simulink model "Cardiovascular"  (Simulink 6.4)
settings: Solver=ode45  StartTime=0.0  StopTime=50  MaxStep=0.01  MinStep=0.0000000000001  RelTol=1e-1
values from neighbouring files (symbols this model uses):
  A = 20.9    [Gas_Exchange_IC.m]    (also in getPneumonia.m = (LF1-LF2)/(1-exp(Rresolve*(t2(end)-t2(1)))))
  B = 92.8    [Gas_Exchange_IC.m]    (also in getPneumonia.m = LungFunction(end)-A)
  C = 10570    [Gas_Exchange_IC.m]
  D = -5.251    [Gas_Exchange_IC.m]
  fcs_max = 47.78    [Cardiovascular_IC.m]    (also in Reflex_Ursino_IC.m)
  fcs_min = 2.52    [Cardiovascular_IC.m]    (also in Reflex_Ursino_IC.m)
  ftbs_min = 0.1    [Cardiovascular_IC.m]    (also in SA_Node_Ursino_IC.m)
  HP_basal = 0.58    [Cardiovascular_IC.m]    (also in SA_Node_Ursino_IC.m)
  k_cs = 11.758    [Cardiovascular_IC.m]    (also in Reflex_Ursino_IC.m)
  Pn = 90    [Cardiovascular_IC.m]    (also in Reflex_Ursino_IC.m)
undefined symbols (not defined in the file or in its folder): Cbp, Cbv, Cep, Cev, Chp, Chv, Cla, Cmp, Cmv, Cpa, Cpp, Cpv, Cra, Csa, Csp, Csv, CvbO2_n, CvhO2_n, CvmO2_n, Dx, ftas_min, Gas_sleep, GbO2, Gbs_sleep, GhO2, GmO2, Gpara_sleep, initx, k_cs_sleep, KElv, KErv, KhCO2, KmCO2, Kr_vc, KRlv, KRrv, ksys, Lpa, Lsa, Mb, Mhn, Mm, P0lv, P0rv, PaCO2_n, Pn_sleep, R_vc_0, Rbpn, Rbv, Rev, Rhpn, Rhv, Rla, Rmv, Rpa, Rpp, Rpv, Rra, Rsa, Rsv ... (+25)
(part 2 of 2)

== system Cardiovascular/Systemic/Systemic  Arteries ==
  Qlv : Inport
  Constant2 : Constant  Value=Vusa  OutDataType=sfix(16)  ConRadixGroup=Use specified scaling  OutScaling=2^0  SampleTime=inf  FramePeriod=inf
  Gain : Gain  Gain=1/Csa  SaturateOnIntegerOverflow=on
  Gain1 : Gain  Orientation=left  Gain=1/Lsa  SaturateOnIntegerOverflow=on
  Gain2 : Gain  Gain=Rsa  SaturateOnIntegerOverflow=on
  Integrator : Integrator  InitialCondition=25.863
  Integrator1 : Integrator  Orientation=left
  SubSystem : Subsystem
  Sum : Sum  Inputs=|+-
  Sum1 : Sum  Inputs=+-  SaturateOnIntegerOverflow=on  InputSameDT=on
  Sum2 : Sum  Inputs=-+-  SaturateOnIntegerOverflow=on  InputSameDT=on
  Qsa : Outport
  tag scope: ABP=global, Vsa=scoped
  wires:
  Sum1/1 -> Integrator/1
  Integrator1/1 -> Gain1/1
  Sum2/1 -> Integrator1/1
  Gain2/1 -> Sum2/3
  Gain1/1 -> Sum1/2, Gain2/1, Qsa/1  "Qsa"
  Integrator/1 -> SubSystem/2(+)
  SubSystem/1(Out) -> Gain/1, [Vsa]
  Constant2/1 -> SubSystem/1(_)
  Qlv/1 -> Sum1/1
  [Psp] -> Sum2/1
  [gPpl] -> Sum/2
  Gain/1 -> Sum/1, [ABP]  "Psa"
  Sum/1 -> Sum2/2

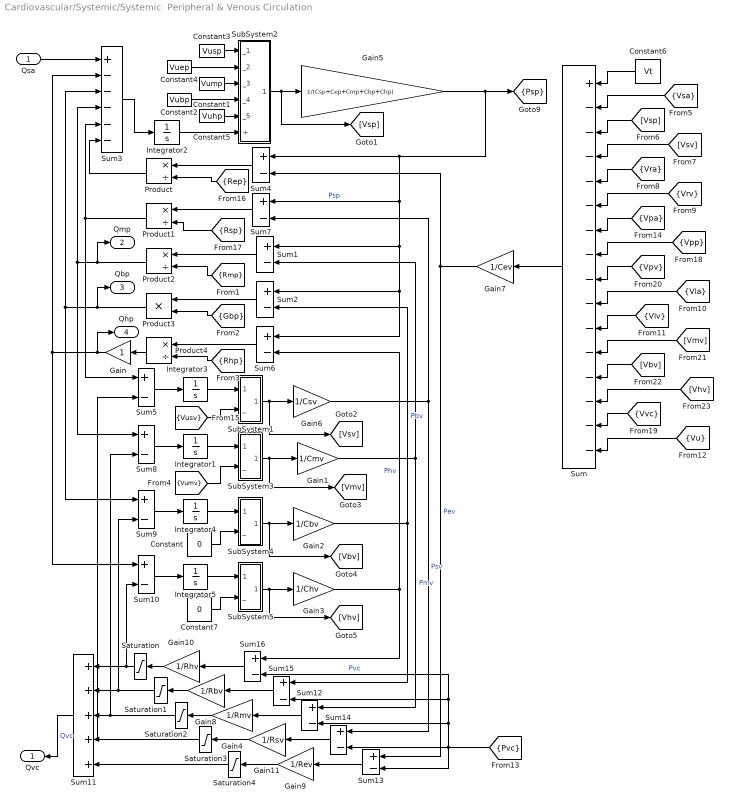
== system Cardiovascular/Systemic/Systemic  Peripheral & Venous Circulation ==
  Qsa : Inport
  Constant : Constant  Value=0  OutDataType=sfix(16)  ConRadixGroup=Use specified scaling  OutScaling=2^0  SampleTime=inf  FramePeriod=inf
  Constant1 : Constant  Value=Vump  OutDataType=sfix(16)  ConRadixGroup=Use specified scaling  OutScaling=2^0  SampleTime=inf  FramePeriod=inf
  Constant2 : Constant  Value=Vubp  OutDataType=sfix(16)  ConRadixGroup=Use specified scaling  OutScaling=2^0  SampleTime=inf  FramePeriod=inf
  Constant3 : Constant  Value=Vusp  OutDataType=sfix(16)  ConRadixGroup=Use specified scaling  OutScaling=2^0  SampleTime=inf  FramePeriod=inf
  Constant4 : Constant  Value=Vuep  OutDataType=sfix(16)  ConRadixGroup=Use specified scaling  OutScaling=2^0  SampleTime=inf  FramePeriod=inf
  Constant5 : Constant  Value=Vuhp  OutDataType=sfix(16)  ConRadixGroup=Use specified scaling  OutScaling=2^0  SampleTime=inf  FramePeriod=inf
  Constant6 : Constant  Orientation=left  Value=Vt  OutDataType=sfix(16)  ConRadixGroup=Use specified scaling  OutScaling=2^0  SampleTime=inf  FramePeriod=inf
  Constant7 : Constant  Value=0  OutDataType=sfix(16)  ConRadixGroup=Use specified scaling  OutScaling=2^0  SampleTime=inf  FramePeriod=inf
  Gain : Gain  Orientation=left
  Gain1 : Gain  Gain=1/Cmv  SaturateOnIntegerOverflow=on
  Gain10 : Gain  Orientation=left  Gain=1/Rhv  SaturateOnIntegerOverflow=on
  Gain11 : Gain  Orientation=left  Gain=1/Rsv  SaturateOnIntegerOverflow=on
  Gain2 : Gain  Gain=1/Cbv  SaturateOnIntegerOverflow=on
  Gain3 : Gain  Gain=1/Chv  SaturateOnIntegerOverflow=on
  Gain4 : Gain  Orientation=left  Gain=1/Rmv  SaturateOnIntegerOverflow=on
  Gain5 : Gain  Gain=1/(Csp+Cep+Cmp+Cbp+Chp)  SaturateOnIntegerOverflow=on
  Gain6 : Gain  Gain=1/Csv  SaturateOnIntegerOverflow=on
  Gain7 : Gain  Orientation=left  Gain=1/Cev  SaturateOnIntegerOverflow=on
  Gain8 : Gain  Orientation=left  Gain=1/Rbv  SaturateOnIntegerOverflow=on
  Gain9 : Gain  Orientation=left  Gain=1/Rev  SaturateOnIntegerOverflow=on
  Integrator{1,3..5} (4 alike) : Integrator
  Integrator2 : Integrator  InitialCondition=Vusp + Vuep+Vump+Vubp+Vuhp
  Product{,1..2,4} (4 alike) : Product  Orientation=left  Inputs=*/  SaturateOnIntegerOverflow=on  RndMeth=Zero  InputSameDT=on
  Product3 : Product  Orientation=left  Inputs=**  SaturateOnIntegerOverflow=on  RndMeth=Zero  InputSameDT=on
  Saturation : Saturate  Orientation=left  UpperLimit=10000  LowerLimit=1
  Saturation1 : Saturate  Orientation=left  UpperLimit=10000  LowerLimit=4
  Saturation2 : Saturate  Orientation=left  UpperLimit=10000  LowerLimit=8
  Saturation3 : Saturate  Orientation=left  UpperLimit=10000  LowerLimit=10
  Saturation4 : Saturate  Orientation=left  UpperLimit=10000  LowerLimit=10
  SubSystem1 : Subsystem
  SubSystem2 : Subsystem
  SubSystem3 : Subsystem
  SubSystem4 : Subsystem
  SubSystem5 : Subsystem
  Sum : Sum  Orientation=left  Inputs=+---------------  SaturateOnIntegerOverflow=on  InputSameDT=on
  Sum{1..2,4,6..7,12..16} (10 alike) : Sum  Orientation=left  Inputs=+-  SaturateOnIntegerOverflow=on  InputSameDT=on
  Sum{5,8..10} (4 alike) : Sum  Inputs=+-  SaturateOnIntegerOverflow=on  InputSameDT=on
  Sum11 : Sum  Orientation=left  Inputs=+++++  SaturateOnIntegerOverflow=on  InputSameDT=on
  Sum3 : Sum  Inputs=+-----  SaturateOnIntegerOverflow=on  InputSameDT=on
  Qvc : Outport  Orientation=left
  Qmp : Outport  Port=2
  Qbp : Outport  Port=3
  Qhp : Outport  Port=4
  tag scope: Psp=scoped
  wires:
  Gain5/1 -> Sum4/1, Sum6/1, Sum2/1, Sum1/1, Sum7/1, [Psp]  "Psp"
  Product1/1 -> Sum3/5, Sum5/1
  Integrator3/1 -> SubSystem1/1(+)
  SubSystem1/1(Out) -> Gain6/1, [Vsv]
  Integrator2/1 -> SubSystem2/6(+)
  SubSystem2/1(Out) -> Gain5/1, [Vsp]
  Sum13/1 -> Gain9/1
  Gain9/1 -> Saturation4/1
  Sum14/1 -> Gain11/1
  [Pvc] -> Sum13/2, Sum14/2, Sum12/2, Sum15/2, Sum16/2  "Pvc"
  Sum5/1 -> Integrator3/1
  Gain11/1 -> Saturation3/1
  [Vusv] -> SubSystem1/2(_)
  Constant3/1 -> SubSystem2/1(_1)
  Constant4/1 -> SubSystem2/2(_2)
  Sum4/1 -> Product/1
  [Rep] -> Product/2
  [Rsp] -> Product1/2
  Sum7/1 -> Product1/1
  Gain6/1 -> Sum7/2, Sum14/1  "Psv"
  Qsa/1 -> Sum3/1
  Gain7/1 -> Sum4/2, Sum13/1  "Pev"
  Sum11/1 -> Qvc/1  "Qvc"
  Sum1/1 -> Product2/1
  [Rmp] -> Product2/2
  Sum2/1 -> Product3/1
  [Gbp] -> Product3/2
  Sum6/1 -> Product4/1
  [Rhp] -> Product4/2
  Product4/1 -> Gain/1
  Product3/1 -> Sum3/3, Sum9/1, Qbp/1
  Product2/1 -> Sum3/4, Sum8/1, Qmp/1
  Product/1 -> Sum3/6
  Constant1/1 -> SubSystem2/3(_3)
  Constant2/1 -> SubSystem2/4(_4)
  Constant5/1 -> SubSystem2/5(_5)
  Sum3/1 -> Integrator2/1
  Integrator1/1 -> SubSystem3/1(+)
  SubSystem3/1(Out) -> Gain1/1, [Vmv]
  Sum8/1 -> Integrator1/1
  [Vumv] -> SubSystem3/2(_)
  Constant6/1 -> Sum/1
  [Vsa] -> Sum/2
  [Vsp] -> Sum/3
  [Vsv] -> Sum/4
  [Vra] -> Sum/5
  [Vrv] -> Sum/6
  [Vpa] -> Sum/7
  [Vpp] -> Sum/8
  [Vpv] -> Sum/9
  [Vla] -> Sum/10
  [Vlv] -> Sum/11
  [Vu] -> Sum/16
  [Vvc] -> Sum/15
  Sum/1 -> Gain7/1
  [Vmv] -> Sum/12
  [Vbv] -> Sum/13
  [Vhv] -> Sum/14
  Integrator4/1 -> SubSystem4/1(+)
  SubSystem4/1(Out) -> Gain2/1, [Vbv]
  Sum9/1 -> Integrator4/1
  Constant/1 -> SubSystem4/2(_)
  Integrator5/1 -> SubSystem5/1(+)
  SubSystem5/1(Out) -> Gain3/1, [Vhv]
  Sum10/1 -> Integrator5/1
  Constant7/1 -> SubSystem5/2(_)
  Gain1/1 -> Sum1/2, Sum12/1  "Pmv"
  Gain2/1 -> Sum2/2, Sum15/1  "Pbv"
  Gain3/1 -> Sum6/2, Sum16/1  "Phv"
  Sum12/1 -> Gain4/1
  Gain4/1 -> Saturation2/1
  Sum15/1 -> Gain8/1
  Gain8/1 -> Saturation1/1
  Sum16/1 -> Gain10/1
  Gain10/1 -> Saturation/1
  Gain/1 -> Sum3/2, Sum10/1, Qhp/1
  Saturation/1 -> Sum11/1, Sum10/2
  Saturation1/1 -> Sum11/2, Sum9/2
  Saturation2/1 -> Sum11/3, Sum8/2
  Saturation3/1 -> Sum11/4, Sum5/2
  Saturation4/1 -> Sum11/5

== system Cardiovascular/Systemic/Vena Cava ==
  Qvc : Inport
  Integrator4 : Integrator
  Product2 : Product  Orientation=left  Inputs=*/  SaturateOnIntegerOverflow=on  RndMeth=Zero  InputSameDT=on
  Pvc : Fcn  Expr=(u>=V_vc_0)*(D1+K1_vc*(u-V_vc_0)) + ( u<V_vc_0)*(D2 + K2_vc*exp(u/V_vc_min))
  Rvc : Fcn  Orientation=left  Expr="Kr_vc * (V_vc_max/u)*  (V_vc_max/u) + R_vc_0"
  Saturation : Saturate  Orientation=left  UpperLimit=10000  LowerLimit=0  ZeroCross=off
  SubSystem3 : Subsystem
  Sum10 : Sum  Inputs=+-  SaturateOnIntegerOverflow=on  InputSameDT=on
  Sum12 : Sum  Orientation=left  Inputs=+-  SaturateOnIntegerOverflow=on  InputSameDT=on
  Sum8 : Sum  Inputs=|++
  V_vc_0 : Constant  Value=130  OutDataType=sfix(16)  ConRadixGroup=Use specified scaling  OutScaling=2^0  SampleTime=inf  FramePeriod=inf
  Qra : Outport  Orientation=left
  tag scope: Pvc=scoped, Vvc=scoped
  wires:
  [gPpl] -> Sum8/2
  Integrator4/1 -> SubSystem3/1(+)
  Sum10/1 -> Integrator4/1
  V_vc_0/1 -> SubSystem3/2(_)
  Pvc/1 -> Sum8/1
  SubSystem3/1(Out) -> Pvc/1, [Vvc]
  Sum8/1 -> [Pvc], Sum12/1
  [Vvc] -> Rvc/1
  [Pra] -> Sum12/2
  Sum12/1 -> Product2/1
  Rvc/1 -> Product2/2
  Product2/1 -> Saturation/1  "Qra"
  Qvc/1 -> Sum10/1
  Saturation/1 -> Sum10/2, Qra/1

== system Cardiovascular/TPR Change/Peri Circ Rep ==
  fes : Inport
  Gas(SI) : Inport  Port=2
  Constant : Constant  Value=ftas_min  OutDataType=sfix(16)  ConRadixGroup=Use specified scaling  OutScaling=2^0  SampleTime=inf  FramePeriod=inf
  Constant1 : Constant  Value=initx(4)  OutDataType=sfix(16)  ConRadixGroup=Use specified scaling  OutScaling=2^0  SampleTime=inf  FramePeriod=inf
  Gain1 : Gain  Gain=0.5  SaturateOnIntegerOverflow=on
  Gain_Rep : Gain  Gain=1.94  SaturateOnIntegerOverflow=on
  Math Function : Math  Operator=log  SaturateOnIntegerOverflow=on
  Product3 : Product  SaturateOnIntegerOverflow=on  InputSameDT=on
  Saturation : Saturate  UpperLimit=inf  LowerLimit=1
  Sum : Sum  Inputs=|+-  SaturateOnIntegerOverflow=on  InputSameDT=on
  Sum1 : Sum  SaturateOnIntegerOverflow=on  InputSameDT=on
  Transfer Fcn : TransferFcn  Denominator=[toux(4) 1]
  Transport Delay : TransportDelay  DelayTime=Dx(4)*0.7  InitialOutput=10  BufferSize=19456
  Rep : Outport
  wires:
  Constant1/1 -> Gain1/1
  Sum1/1 -> Rep/1
  Transfer Fcn/1 -> Sum1/1
  Math Function/1 -> Gain_Rep/1
  Saturation/1 -> Math Function/1
  Sum/1 -> Saturation/1
  Constant/1 -> Sum/2
  Transport Delay/1 -> Sum/1
  fes/1 -> Transport Delay/1
  Gas(SI)/1 -> Product3/2
  Gain_Rep/1 -> Product3/1
  Product3/1 -> Transfer Fcn/1
  Gain1/1 -> Sum1/2

== system Cardiovascular/TPR Change/Peri Circ Rmp ==
  fes : Inport
  Gas(SI) : Inport  Port=2
  Constant : Constant  Value=ftas_min  OutDataType=sfix(16)  ConRadixGroup=Use specified scaling  OutScaling=2^0  SampleTime=inf  FramePeriod=inf
  Constant1 : Constant  Value=initx(10)  OutDataType=sfix(16)  ConRadixGroup=Use specified scaling  OutScaling=2^0  SampleTime=inf  FramePeriod=inf
  Gain1 : Gain  Orientation=up  Gain=0.5  SaturateOnIntegerOverflow=on
  Gain_Rmp : Gain  Gain=2.47  SaturateOnIntegerOverflow=on
  Math Function : Math  Operator=log  SaturateOnIntegerOverflow=on
  Product3 : Product  SaturateOnIntegerOverflow=on  InputSameDT=on
  Saturation : Saturate  UpperLimit=inf  LowerLimit=1
  Sum : Sum  Inputs=+-  SaturateOnIntegerOverflow=on  InputSameDT=on
  Sum1 : Sum  SaturateOnIntegerOverflow=on  InputSameDT=on
  Transfer Fcn : TransferFcn  Denominator=[toux(10) 1]
  Transport Delay : TransportDelay  DelayTime=Dx(10)*0.7  InitialOutput=10  BufferSize=19456
  Rmp_n : Outport
  wires:
  Constant1/1 -> Gain1/1
  Sum1/1 -> Rmp_n/1
  Transfer Fcn/1 -> Sum1/1
  Math Function/1 -> Gain_Rmp/1
  Saturation/1 -> Math Function/1
  Sum/1 -> Saturation/1
  Constant/1 -> Sum/2
  Transport Delay/1 -> Sum/1
  fes/1 -> Transport Delay/1
  Gas(SI)/1 -> Product3/2
  Gain_Rmp/1 -> Product3/1
  Product3/1 -> Transfer Fcn/1
  Gain1/1 -> Sum1/2

== system Cardiovascular/TPR Change/Peri Circ Rsp ==
  fes : Inport
  Gas(SI) : Inport  Port=2
  Constant : Constant  Value=ftas_min  OutDataType=sfix(16)  ConRadixGroup=Use specified scaling  OutScaling=2^0  SampleTime=inf  FramePeriod=inf
  Constant1 : Constant  Value=initx(3)  OutDataType=sfix(16)  ConRadixGroup=Use specified scaling  OutScaling=2^0  SampleTime=inf  FramePeriod=inf
  Gain : Gain  Gain=0.5  SaturateOnIntegerOverflow=on
  Gain_Rsp : Gain  Gain=0.695  SaturateOnIntegerOverflow=on
  Math Function : Math  Operator=log  SaturateOnIntegerOverflow=on
  Product3 : Product  SaturateOnIntegerOverflow=on  InputSameDT=on
  Saturation : Saturate  UpperLimit=inf  LowerLimit=1
  Sum : Sum  Inputs=+-  SaturateOnIntegerOverflow=on  InputSameDT=on
  Sum1 : Sum  SaturateOnIntegerOverflow=on  InputSameDT=on
  Transfer Fcn : TransferFcn  Denominator=[toux(3) 1]
  Transport Delay : TransportDelay  DelayTime=Dx(3)*0.7  InitialOutput=10  BufferSize=19456
  Rsp : Outport
  wires:
  fes/1 -> Transport Delay/1
  Transport Delay/1 -> Sum/1
  Constant/1 -> Sum/2
  Sum/1 -> Saturation/1
  Saturation/1 -> Math Function/1
  Math Function/1 -> Gain_Rsp/1
  Transfer Fcn/1 -> Sum1/1
  Sum1/1 -> Rsp/1
  Constant1/1 -> Gain/1
  Gas(SI)/1 -> Product3/2
  Gain_Rsp/1 -> Product3/1
  Product3/1 -> Transfer Fcn/1
  Gain/1 -> Sum1/2

== system Cardiovascular/TPR Change/Saving TPR ==
  In1 : Inport
  Clock : Clock
      settings: Decimation=10
  Gain : Gain  Gain=1/(3600*24*7)
  Rounding Function : Rounding
  Switch Case : SwitchCase  CaseConditions={0,1,2,3,4,5,6,7,8}  SampleTime=0.1
  Switch Case Action Subsystem : Subsystem  TreatAsAtomicUnit=on
  Switch Case Action Subsystem1 : Subsystem  TreatAsAtomicUnit=on
  Switch Case Action Subsystem2 : Subsystem  TreatAsAtomicUnit=on
  Switch Case Action Subsystem3 : Subsystem  TreatAsAtomicUnit=on
  Switch Case Action Subsystem4 : Subsystem  TreatAsAtomicUnit=on
  Switch Case Action Subsystem5 : Subsystem  TreatAsAtomicUnit=on
  Switch Case Action Subsystem6 : Subsystem  TreatAsAtomicUnit=on
  Switch Case Action Subsystem7 : Subsystem  TreatAsAtomicUnit=on
  Switch Case Action Subsystem8 : Subsystem  TreatAsAtomicUnit=on
  Switch Case Action Subsystem9 : Subsystem  TreatAsAtomicUnit=on
  wires:
  Clock/1 -> Gain/1
  Switch Case/1 -> Switch Case Action Subsystem/Action
  Switch Case/2 -> Switch Case Action Subsystem1/Action
  Switch Case/3 -> Switch Case Action Subsystem2/Action
  Switch Case/10 -> Switch Case Action Subsystem3/Action
  Rounding Function/1 -> Switch Case/1
  In1/1 -> Switch Case Action Subsystem/1(In1), Switch Case Action Subsystem1/1(In1), Switch Case Action Subsystem2/1(In1), Switch Case Action Subsystem5/1(In1), Switch Case Action Subsystem3/1(In1), Switch Case Action Subsystem9/1(In1), Switch Case Action Subsystem8/1(In1), Switch Case Action Subsystem7/1(In1), Switch Case Action Subsystem6/1(In1), Switch Case Action Subsystem4/1(In1)
  Gain/1 -> Rounding Function/1
  Switch Case/4 -> Switch Case Action Subsystem4/Action
  Switch Case/5 -> Switch Case Action Subsystem5/Action
  Switch Case/6 -> Switch Case Action Subsystem6/Action
  Switch Case/7 -> Switch Case Action Subsystem7/Action
  Switch Case/8 -> Switch Case Action Subsystem8/Action
  Switch Case/9 -> Switch Case Action Subsystem9/Action

== system Cardiovascular/TPR Change/Venous Circ Vuev ==
  fes : Inport
  Gas(SI) : Inport  Port=2
  Constant : Constant  Value=ftas_min  OutDataType=sfix(16)  ConRadixGroup=Use specified scaling  OutScaling=2^0  SampleTime=inf  FramePeriod=inf
  Constant1 : Constant  Value=initx(6)  OutDataType=sfix(16)  ConRadixGroup=Use specified scaling  OutScaling=2^0  SampleTime=inf  FramePeriod=inf
  Divide : Product  Inputs=**  OutScaling=2^-10
  Gain_Vuev : Gain  Gain=-74.21  SaturateOnIntegerOverflow=on
  Math Function : Math  Operator=log  SaturateOnIntegerOverflow=on
  Saturation : Saturate  UpperLimit=inf  LowerLimit=1
  Sum : Sum  Inputs=|+-  SaturateOnIntegerOverflow=on  InputSameDT=on
  Sum1 : Sum  SaturateOnIntegerOverflow=on  InputSameDT=on
  Transfer Fcn : TransferFcn  Denominator=[toux(6)*0.7 1]
  Transport Delay : TransportDelay  DelayTime=Dx(6)*0.7  InitialOutput=10  BufferSize=19456
  Vuev : Outport
  wires:
  Constant1/1 -> Sum1/2
  Sum1/1 -> Vuev/1
  Transfer Fcn/1 -> Sum1/1
  Math Function/1 -> Gain_Vuev/1
  Saturation/1 -> Math Function/1
  Sum/1 -> Saturation/1
  Constant/1 -> Sum/2
  Transport Delay/1 -> Sum/1
  fes/1 -> Transport Delay/1
  Gain_Vuev/1 -> Divide/1
  Divide/1 -> Transfer Fcn/1
  Gas(SI)/1 -> Divide/2

== system Cardiovascular/TPR Change/Venous Circ Vumv ==
  fes : Inport
  Gas(SI) : Inport  Port=2
  Constant : Constant  Value=ftas_min  OutDataType=sfix(16)  ConRadixGroup=Use specified scaling  OutScaling=2^0  SampleTime=inf  FramePeriod=inf
  Constant1 : Constant  Value=initx(9)  OutDataType=sfix(16)  ConRadixGroup=Use specified scaling  OutScaling=2^0  SampleTime=inf  FramePeriod=inf
  Divide : Product  Inputs=**  OutScaling=2^-10
  Gain_Vumv : Gain  Gain=-58.29  SaturateOnIntegerOverflow=on
  Math Function : Math  Operator=log  SaturateOnIntegerOverflow=on
  Saturation : Saturate  UpperLimit=inf  LowerLimit=1
  Sum : Sum  Inputs=+-  SaturateOnIntegerOverflow=on  InputSameDT=on
  Sum1 : Sum  SaturateOnIntegerOverflow=on  InputSameDT=on
  Transfer Fcn : TransferFcn  Denominator=[toux(9)*0.7 1]
  Transport Delay : TransportDelay  DelayTime=Dx(9)*0.7  InitialOutput=10  BufferSize=19456
  Vumv : Outport
  wires:
  Constant1/1 -> Sum1/2
  Sum1/1 -> Vumv/1
  Transfer Fcn/1 -> Sum1/1
  Math Function/1 -> Gain_Vumv/1
  Saturation/1 -> Math Function/1
  Sum/1 -> Saturation/1
  Constant/1 -> Sum/2
  Transport Delay/1 -> Sum/1
  fes/1 -> Transport Delay/1
  Gas(SI)/1 -> Divide/2
  Gain_Vumv/1 -> Divide/1
  Divide/1 -> Transfer Fcn/1

== system Cardiovascular/TPR Change/Venous Circ Vusv ==
  fes : Inport
  Gas(SI) : Inport  Port=2
  Constant : Constant  Value=ftas_min  OutDataType=sfix(16)  ConRadixGroup=Use specified scaling  OutScaling=2^0  SampleTime=inf  FramePeriod=inf
  Constant1 : Constant  Value=initx(5)  OutDataType=sfix(16)  ConRadixGroup=Use specified scaling  OutScaling=2^0  SampleTime=inf  FramePeriod=inf
  Divide : Product  Inputs=**  OutScaling=2^-10
  Gain_Vusv : Gain  Gain=-265.4  SaturateOnIntegerOverflow=on
  Math Function : Math  Operator=log  SaturateOnIntegerOverflow=on
  Saturation : Saturate  UpperLimit=inf  LowerLimit=1
  Sum : Sum  Inputs=|+-  SaturateOnIntegerOverflow=on  InputSameDT=on
  Sum1 : Sum  SaturateOnIntegerOverflow=on  InputSameDT=on
  Transfer Fcn : TransferFcn  Denominator=[toux(5)*0.7 1]
  Transport Delay : TransportDelay  DelayTime=Dx(5)*0.7  InitialOutput=10  BufferSize=19456
  Vusv : Outport
  wires:
  fes/1 -> Transport Delay/1
  Transport Delay/1 -> Sum/1
  Constant/1 -> Sum/2
  Sum/1 -> Saturation/1
  Saturation/1 -> Math Function/1
  Math Function/1 -> Gain_Vusv/1
  Transfer Fcn/1 -> Sum1/1
  Sum1/1 -> Vusv/1
  Constant1/1 -> Sum1/2
  Gas(SI)/1 -> Divide/2
  Gain_Vusv/1 -> Divide/1
  Divide/1 -> Transfer Fcn/1

== system Cardiovascular/Left Heart/Saving PVleft/Switch Case Action Subsystem ==
  In1 : Inport
  Action Port : ActionPort
  To File : ToFile  Filename=PVleft1.mat  MatrixName=PLeft_VLeft  SampleTime=0.1
  wires:
  In1/1 -> To File/1

== system Cardiovascular/Left Heart/Saving PVleft/Switch Case Action Subsystem1 ==
  In1 : Inport
  Action Port : ActionPort
  To File : ToFile  Filename=PVleft2.mat  MatrixName=PLeft_VLeft  SampleTime=0.1
  wires:
  In1/1 -> To File/1

== system Cardiovascular/Left Heart/Saving PVleft/Switch Case Action Subsystem2 ==
  In1 : Inport
  Action Port : ActionPort
  To File : ToFile  Filename=PVleft3.mat  MatrixName=PLeft_VLeft  SampleTime=0.1
  wires:
  In1/1 -> To File/1

== system Cardiovascular/Left Heart/Saving PVleft/Switch Case Action Subsystem3 ==
  In1 : Inport
  Action Port : ActionPort
  To File : ToFile  Filename=PVleft10.mat  MatrixName=PLeft_VLeft  SampleTime=0.1
  wires:
  In1/1 -> To File/1

== system Cardiovascular/Left Heart/Saving PVleft/Switch Case Action Subsystem4 ==
  In1 : Inport
  Action Port : ActionPort
  To File : ToFile  Filename=PVleft4.mat  MatrixName=PLeft_VLeft  SampleTime=0.1
  wires:
  In1/1 -> To File/1

== system Cardiovascular/Left Heart/Saving PVleft/Switch Case Action Subsystem5 ==
  In1 : Inport
  Action Port : ActionPort
  To File : ToFile  Filename=PVleft5.mat  MatrixName=PLeft_VLeft  SampleTime=0.1
  wires:
  In1/1 -> To File/1

== system Cardiovascular/Left Heart/Saving PVleft/Switch Case Action Subsystem6 ==
  In1 : Inport
  Action Port : ActionPort
  To File : ToFile  Filename=PVleft6.mat  MatrixName=PLeft_VLeft  SampleTime=0.1
  wires:
  In1/1 -> To File/1

== system Cardiovascular/Left Heart/Saving PVleft/Switch Case Action Subsystem7 ==
  In1 : Inport
  Action Port : ActionPort
  To File : ToFile  Filename=PVleft7.mat  MatrixName=PLeft_VLeft  SampleTime=0.1
  wires:
  In1/1 -> To File/1

== system Cardiovascular/Left Heart/Saving PVleft/Switch Case Action Subsystem8 ==
  In1 : Inport
  Action Port : ActionPort
  To File : ToFile  Filename=PVleft8.mat  MatrixName=PLeft_VLeft  SampleTime=0.1
  wires:
  In1/1 -> To File/1

== system Cardiovascular/Left Heart/Saving PVleft/Switch Case Action Subsystem9 ==
  In1 : Inport
  Action Port : ActionPort
  To File : ToFile  Filename=PVleft9.mat  MatrixName=PLeft_VLeft  SampleTime=0.1
  wires:
  In1/1 -> To File/1

== system Cardiovascular/Local Flow Regulation/Cerebral Circulation Regulation/Subsystem ==
  QbpIC : Inport
  If : If  IfExpression=u1 == 0  ShowElse=off
  If Action Subsystem : Subsystem  TreatAsAtomicUnit=on
  Step 10sec : Step  Time=0  After=5  SampleTime=0
  Step1 : Step  Time=5  After=-5  SampleTime=0
  Sum : Sum  Inputs=|++
  Sum1 : Sum  Inputs=|++
  Qbp : Outport
  wires:
  Step 10sec/1 -> Sum/1
  Step1/1 -> Sum/2
  Sum/1 -> Sum1/2, If/1
  If/1 -> If Action Subsystem/Action
  QbpIC/1 -> If Action Subsystem/1(In1)
  Sum1/1 -> Qbp/1
  If Action Subsystem/1(Out1) -> Sum1/1

== system Cardiovascular/Local Flow Regulation/Coronary Circulation Regulation2/Subsystem ==
  Q : Inport
  If : If  IfExpression=u1 == 0  ShowElse=off
  If Action Subsystem : Subsystem  TreatAsAtomicUnit=on
  Step 10sec : Step  Time=0  SampleTime=0
  Step1 : Step  After=-1  SampleTime=0
  Sum : Sum  Inputs=|++
  Sum1 : Sum  Inputs=|++
  Qhp : Outport
  wires:
  Step 10sec/1 -> Sum/1
  Step1/1 -> Sum/2
  Sum/1 -> Sum1/2, If/1
  If/1 -> If Action Subsystem/Action
  Q/1 -> If Action Subsystem/1(In1)
  Sum1/1 -> Qhp/1
  If Action Subsystem/1(Out1) -> Sum1/1

== system Cardiovascular/Local Flow Regulation/Muscular Circulation Regulation1/Subsystem ==
  Q : Inport
  If : If  IfExpression=u1 == 0  ShowElse=off
  If Action Subsystem : Subsystem  TreatAsAtomicUnit=on
  Step 10sec : Step  Time=0  After=5  SampleTime=0
  Step1 : Step  After=-5  SampleTime=0
  Sum : Sum  Inputs=|++
  Sum1 : Sum  Inputs=|++
  Qmp : Outport
  wires:
  Step 10sec/1 -> Sum/1
  Step1/1 -> Sum/2
  Sum/1 -> Sum1/2, If/1
  If/1 -> If Action Subsystem/Action
  Q/1 -> If Action Subsystem/1(In1)
  Sum1/1 -> Qmp/1
  If Action Subsystem/1(Out1) -> Sum1/1

== system Cardiovascular/SA-node and Autonomic Control/Left Ventricle/SubSystem1 ==
  _ : Inport
  + : Inport  Port=2
  Saturation : Saturate  UpperLimit=10000  LowerLimit=0
  Sum : Sum  Inputs=|-+  SaturateOnIntegerOverflow=on  InputSameDT=on
  Out : Outport
  wires:
  _/1 -> Sum/1
  +/1 -> Sum/2
  Sum/1 -> Saturation/1
  Saturation/1 -> Out/1

== system Cardiovascular/SA-node and Autonomic Control/RR Interval/If Action Subsystem ==
  In1 : Inport
  Action Port : ActionPort
  Out1 : Outport
  wires:
  In1/1 -> Out1/1

== system Cardiovascular/SA-node and Autonomic Control/RR Interval/Saving varHeartPeriod ==
  In1 : Inport
  Clock : Clock
      settings: Decimation=10
  Gain : Gain  Gain=1/(3600*24*7)
  Rounding Function : Rounding
  Switch Case : SwitchCase  CaseConditions={0,1,2,3,4,5,6,7,8}  SampleTime=0.1
  Switch Case Action Subsystem : Subsystem  TreatAsAtomicUnit=on
  Switch Case Action Subsystem1 : Subsystem  TreatAsAtomicUnit=on
  Switch Case Action Subsystem2 : Subsystem  TreatAsAtomicUnit=on
  Switch Case Action Subsystem3 : Subsystem  TreatAsAtomicUnit=on
  Switch Case Action Subsystem4 : Subsystem  TreatAsAtomicUnit=on
  Switch Case Action Subsystem5 : Subsystem  TreatAsAtomicUnit=on
  Switch Case Action Subsystem6 : Subsystem  TreatAsAtomicUnit=on
  Switch Case Action Subsystem7 : Subsystem  TreatAsAtomicUnit=on
  Switch Case Action Subsystem8 : Subsystem  TreatAsAtomicUnit=on
  Switch Case Action Subsystem9 : Subsystem  TreatAsAtomicUnit=on
  wires:
  Clock/1 -> Gain/1
  Switch Case/1 -> Switch Case Action Subsystem/Action
  Switch Case/2 -> Switch Case Action Subsystem1/Action
  Switch Case/3 -> Switch Case Action Subsystem2/Action
  Switch Case/10 -> Switch Case Action Subsystem3/Action
  Rounding Function/1 -> Switch Case/1
  In1/1 -> Switch Case Action Subsystem/1(In1), Switch Case Action Subsystem1/1(In1), Switch Case Action Subsystem2/1(In1), Switch Case Action Subsystem5/1(In1), Switch Case Action Subsystem3/1(In1), Switch Case Action Subsystem9/1(In1), Switch Case Action Subsystem8/1(In1), Switch Case Action Subsystem7/1(In1), Switch Case Action Subsystem6/1(In1), Switch Case Action Subsystem4/1(In1)
  Gain/1 -> Rounding Function/1
  Switch Case/4 -> Switch Case Action Subsystem4/Action
  Switch Case/5 -> Switch Case Action Subsystem5/Action
  Switch Case/6 -> Switch Case Action Subsystem6/Action
  Switch Case/7 -> Switch Case Action Subsystem7/Action
  Switch Case/8 -> Switch Case Action Subsystem8/Action
  Switch Case/9 -> Switch Case Action Subsystem9/Action

== system Cardiovascular/SA-node and Autonomic Control/Right Ventricle/SubSystem1 ==
  _ : Inport
  + : Inport  Port=2
  Saturation : Saturate  UpperLimit=10000  LowerLimit=0
  Sum : Sum  Inputs=|-+  SaturateOnIntegerOverflow=on  InputSameDT=on
  Out : Outport
  wires:
  Saturation/1 -> Out/1
  Sum/1 -> Saturation/1
  +/1 -> Sum/2
  _/1 -> Sum/1

== system Cardiovascular/SA-node and Autonomic Control/phi/SubSystem ==
  In1 : Inport
  Trigger : TriggerPort
  Data Store Write : DataStoreWrite  DataStoreName=A  SampleTime=-1
  wires:
  In1/1 -> Data Store Write/1

== system Cardiovascular/Systemic/Systemic  Arteries/SubSystem ==
  _ : Inport
  + : Inport  Port=2
  Saturation : Saturate  UpperLimit=10000  LowerLimit=0
  Sum : Sum  Inputs=|-+  SaturateOnIntegerOverflow=on  InputSameDT=on
  Out : Outport
  wires:
  _/1 -> Sum/1
  +/1 -> Sum/2
  Sum/1 -> Saturation/1
  Saturation/1 -> Out/1

== system Cardiovascular/Systemic/Systemic  Peripheral & Venous Circulation/SubSystem1 ==
  + : Inport
  _ : Inport  Port=2
  Saturation : Saturate  UpperLimit=10000  LowerLimit=0
  Sum : Sum  Inputs=|+-  SaturateOnIntegerOverflow=on  InputSameDT=on
  Out : Outport
  wires:
  Saturation/1 -> Out/1
  Sum/1 -> Saturation/1
  _/1 -> Sum/2
  +/1 -> Sum/1

== system Cardiovascular/Systemic/Systemic  Peripheral & Venous Circulation/SubSystem2 ==
  _1 : Inport
  _2 : Inport  Port=2
  _3 : Inport  Port=3
  _4 : Inport  Port=4
  _5 : Inport  Port=5
  + : Inport  Port=6
  Saturation : Saturate  UpperLimit=10000  LowerLimit=0  ZeroCross=off
  Sum : Sum  Inputs=|-----+  SaturateOnIntegerOverflow=on  InputSameDT=on
  Out : Outport
  wires:
  Saturation/1 -> Out/1
  Sum/1 -> Saturation/1
  _1/1 -> Sum/1
  _2/1 -> Sum/2
  _3/1 -> Sum/3
  _4/1 -> Sum/4
  _5/1 -> Sum/5
  +/1 -> Sum/6

== system Cardiovascular/Systemic/Systemic  Peripheral & Venous Circulation/SubSystem3 ==
  + : Inport
  _ : Inport  Port=2
  Saturation : Saturate  UpperLimit=10000  LowerLimit=0
  Sum : Sum  Inputs=|+-  SaturateOnIntegerOverflow=on  InputSameDT=on
  Out : Outport
  wires:
  Saturation/1 -> Out/1
  Sum/1 -> Saturation/1
  _/1 -> Sum/2
  +/1 -> Sum/1

== system Cardiovascular/Systemic/Systemic  Peripheral & Venous Circulation/SubSystem4 ==
  + : Inport
  _ : Inport  Port=2
  Saturation : Saturate  UpperLimit=10000  LowerLimit=0
  Sum : Sum  Inputs=|+-  SaturateOnIntegerOverflow=on  InputSameDT=on
  Out : Outport
  wires:
  Saturation/1 -> Out/1
  Sum/1 -> Saturation/1
  _/1 -> Sum/2
  +/1 -> Sum/1

== system Cardiovascular/Systemic/Systemic  Peripheral & Venous Circulation/SubSystem5 ==
  + : Inport
  _ : Inport  Port=2
  Saturation : Saturate  UpperLimit=10000  LowerLimit=0
  Sum : Sum  Inputs=|+-  SaturateOnIntegerOverflow=on  InputSameDT=on
  Out : Outport
  wires:
  Saturation/1 -> Out/1
  Sum/1 -> Saturation/1
  _/1 -> Sum/2
  +/1 -> Sum/1

== system Cardiovascular/Systemic/Vena Cava/SubSystem3 ==
  + : Inport
  _ : Inport  Port=2
  Saturation : Saturate  UpperLimit=10000  LowerLimit=0
  Sum : Sum  Inputs=|+-  SaturateOnIntegerOverflow=on  InputSameDT=on
  Out : Outport
  wires:
  Saturation/1 -> Out/1
  Sum/1 -> Saturation/1
  _/1 -> Sum/2
  +/1 -> Sum/1

== system Cardiovascular/TPR Change/Saving TPR/Switch Case Action Subsystem ==
  In1 : Inport
  Action Port : ActionPort
  To File : ToFile  Filename=TPR1.mat  MatrixName=TPR  SampleTime=0.1
  wires:
  In1/1 -> To File/1

== system Cardiovascular/TPR Change/Saving TPR/Switch Case Action Subsystem1 ==
  In1 : Inport
  Action Port : ActionPort
  To File : ToFile  Filename=TPR2.mat  MatrixName=TPR  SampleTime=0.1
  wires:
  In1/1 -> To File/1

== system Cardiovascular/TPR Change/Saving TPR/Switch Case Action Subsystem2 ==
  In1 : Inport
  Action Port : ActionPort
  To File : ToFile  Filename=TPR3.mat  MatrixName=TPR  SampleTime=0.1
  wires:
  In1/1 -> To File/1

== system Cardiovascular/TPR Change/Saving TPR/Switch Case Action Subsystem3 ==
  In1 : Inport
  Action Port : ActionPort
  To File : ToFile  Filename=TPR10.mat  MatrixName=TPR  SampleTime=0.1
  wires:
  In1/1 -> To File/1

== system Cardiovascular/TPR Change/Saving TPR/Switch Case Action Subsystem4 ==
  In1 : Inport
  Action Port : ActionPort
  To File : ToFile  Filename=TPR4.mat  MatrixName=TPR  SampleTime=0.1
  wires:
  In1/1 -> To File/1

== system Cardiovascular/TPR Change/Saving TPR/Switch Case Action Subsystem5 ==
  In1 : Inport
  Action Port : ActionPort
  To File : ToFile  Filename=TPR5.mat  MatrixName=TPR  SampleTime=0.1
  wires:
  In1/1 -> To File/1

== system Cardiovascular/TPR Change/Saving TPR/Switch Case Action Subsystem6 ==
  In1 : Inport
  Action Port : ActionPort
  To File : ToFile  Filename=TPR6.mat  MatrixName=TPR  SampleTime=0.1
  wires:
  In1/1 -> To File/1

== system Cardiovascular/TPR Change/Saving TPR/Switch Case Action Subsystem7 ==
  In1 : Inport
  Action Port : ActionPort
  To File : ToFile  Filename=TPR7.mat  MatrixName=TPR  SampleTime=0.1
  wires:
  In1/1 -> To File/1

== system Cardiovascular/TPR Change/Saving TPR/Switch Case Action Subsystem8 ==
  In1 : Inport
  Action Port : ActionPort
  To File : ToFile  Filename=TPR8.mat  MatrixName=TPR  SampleTime=0.1
  wires:
  In1/1 -> To File/1

== system Cardiovascular/TPR Change/Saving TPR/Switch Case Action Subsystem9 ==
  In1 : Inport
  Action Port : ActionPort
  To File : ToFile  Filename=TPR9.mat  MatrixName=TPR  SampleTime=0.1
  wires:
  In1/1 -> To File/1

== system Cardiovascular/Local Flow Regulation/Cerebral Circulation Regulation/Subsystem/If Action Subsystem ==
  In1 : Inport
  Action Port : ActionPort
  Out1 : Outport
  wires:
  In1/1 -> Out1/1

== system Cardiovascular/Local Flow Regulation/Coronary Circulation Regulation2/Subsystem/If Action Subsystem ==
  In1 : Inport
  Action Port : ActionPort
  Out1 : Outport
  wires:
  In1/1 -> Out1/1

== system Cardiovascular/Local Flow Regulation/Muscular Circulation Regulation1/Subsystem/If Action Subsystem ==
  In1 : Inport
  Action Port : ActionPort
  Out1 : Outport
  wires:
  In1/1 -> Out1/1

== system Cardiovascular/SA-node and Autonomic Control/RR Interval/Saving varHeartPeriod/Switch Case Action Subsystem ==
  In1 : Inport
  Action Port : ActionPort
  To File : ToFile  Filename=varHeartPeriod1.mat  MatrixName=HPsa_HPin_HPout_HP_Enable  SampleTime=0.1
  wires:
  In1/1 -> To File/1

== system Cardiovascular/SA-node and Autonomic Control/RR Interval/Saving varHeartPeriod/Switch Case Action Subsystem1 ==
  In1 : Inport
  Action Port : ActionPort
  To File : ToFile  Filename=varHeartPeriod2.mat  MatrixName=HPsa_HPin_HPout_HP_Enable  SampleTime=0.1
  wires:
  In1/1 -> To File/1

== system Cardiovascular/SA-node and Autonomic Control/RR Interval/Saving varHeartPeriod/Switch Case Action Subsystem2 ==
  In1 : Inport
  Action Port : ActionPort
  To File : ToFile  Filename=varHeartPeriod3.mat  MatrixName=HPsa_HPin_HPout_HP_Enable  SampleTime=0.1
  wires:
  In1/1 -> To File/1

== system Cardiovascular/SA-node and Autonomic Control/RR Interval/Saving varHeartPeriod/Switch Case Action Subsystem3 ==
  In1 : Inport
  Action Port : ActionPort
  To File : ToFile  Filename=varHeartPeriod10.mat  MatrixName=HPsa_HPin_HPout_HP_Enable  SampleTime=0.1
  wires:
  In1/1 -> To File/1

== system Cardiovascular/SA-node and Autonomic Control/RR Interval/Saving varHeartPeriod/Switch Case Action Subsystem4 ==
  In1 : Inport
  Action Port : ActionPort
  To File : ToFile  Filename=varHeartPeriod4.mat  MatrixName=HPsa_HPin_HPout_HP_Enable  SampleTime=0.1
  wires:
  In1/1 -> To File/1

== system Cardiovascular/SA-node and Autonomic Control/RR Interval/Saving varHeartPeriod/Switch Case Action Subsystem5 ==
  In1 : Inport
  Action Port : ActionPort
  To File : ToFile  Filename=varHeartPeriod5.mat  MatrixName=HPsa_HPin_HPout_HP_Enable  SampleTime=0.1
  wires:
  In1/1 -> To File/1

== system Cardiovascular/SA-node and Autonomic Control/RR Interval/Saving varHeartPeriod/Switch Case Action Subsystem6 ==
  In1 : Inport
  Action Port : ActionPort
  To File : ToFile  Filename=varHeartPeriod6.mat  MatrixName=HPsa_HPin_HPout_HP_Enable  SampleTime=0.1
  wires:
  In1/1 -> To File/1

== system Cardiovascular/SA-node and Autonomic Control/RR Interval/Saving varHeartPeriod/Switch Case Action Subsystem7 ==
  In1 : Inport
  Action Port : ActionPort
  To File : ToFile  Filename=varHeartPeriod7.mat  MatrixName=HPsa_HPin_HPout_HP_Enable  SampleTime=0.1
  wires:
  In1/1 -> To File/1

== system Cardiovascular/SA-node and Autonomic Control/RR Interval/Saving varHeartPeriod/Switch Case Action Subsystem8 ==
  In1 : Inport
  Action Port : ActionPort
  To File : ToFile  Filename=varHeartPeriod8.mat  MatrixName=HPsa_HPin_HPout_HP_Enable  SampleTime=0.1
  wires:
  In1/1 -> To File/1

== system Cardiovascular/SA-node and Autonomic Control/RR Interval/Saving varHeartPeriod/Switch Case Action Subsystem9 ==
  In1 : Inport
  Action Port : ActionPort
  To File : ToFile  Filename=varHeartPeriod9.mat  MatrixName=HPsa_HPin_HPout_HP_Enable  SampleTime=0.1
  wires:
  In1/1 -> To File/1
